simulink model "hikaku"  (R2018b)
settings: Solver=VariableStepAuto  StartTime=0.0  StopTime=3  RelTol=1e-3
values from neighbouring files (symbols this model uses):
  K = lqr(sys_A, sys_B, Q, R)    [LQRadjuster.m]
  L = [0.25; 0.75; -0.15; 0.35]    [LQRadjuster.m]
  x0 = [20*pi/180;0;0;0]    [LQRadjuster.m]
undefined symbols (not defined in the file or in its folder): sys_Ad, sys_Bd, sys_C, sys_D, Ts
settings Model: Creator=kuwano  LastModifiedBy=kuwano

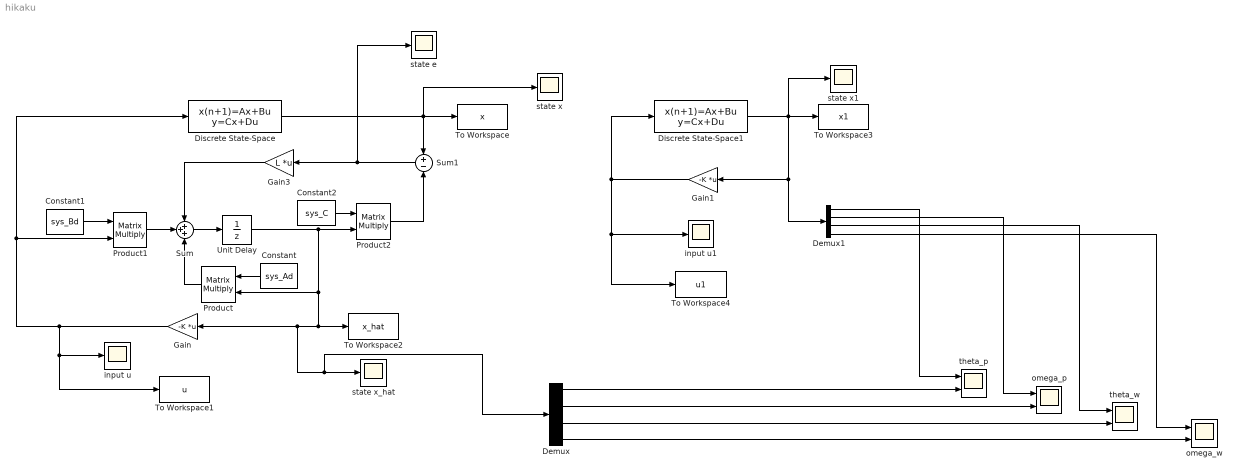
== system hikaku ==
  Constant : Constant  Value=sys_Ad  VectorParams1D=off
  Constant1 : Constant  Value=sys_Bd  VectorParams1D=off
  Constant2 : Constant  Value=sys_C  VectorParams1D=off
  Demux : Demux
  Demux1 : Demux
  Discrete State-Space : DiscreteStateSpace  A=sys_Ad  B=sys_Bd  C=sys_C  D=sys_D  InitialCondition=x0  SampleTime=Ts
  Discrete State-Space1 : DiscreteStateSpace  A=sys_Ad  B=sys_Bd  C=eye(4)  D=[0; 0; 0; 0]  InitialCondition=x0  SampleTime=Ts
  Gain : Gain  Gain=-K  Multiplication=Matrix(K*u)
  Gain1 : Gain  Gain=-K  Multiplication=Matrix(K*u)
  Gain3 : Gain  Gain=L  Multiplication=Matrix(K*u)
  Product : Product  Multiplication=Matrix(*)
  Product1 : Product  Multiplication=Matrix(*)
  Product2 : Product  Multiplication=Matrix(*)
  Sum : Sum  Inputs=+++
  Sum1 : Sum  Inputs=+|-
  To Workspace : ToWorkspace  VariableName=x  SampleTime=-1
  To Workspace1 : ToWorkspace  VariableName=u  SampleTime=-1
  To Workspace2 : ToWorkspace  VariableName=x_hat  SampleTime=-1
  To Workspace3 : ToWorkspace  VariableName=x1  SampleTime=-1
  To Workspace4 : ToWorkspace  VariableName=u1  SampleTime=-1
  Unit Delay : UnitDelay  InitialCondition=[0; 0; 0; 0]  SampleTime=-1
  input u : Scope
  input u1 : Scope
  omega_p : Scope  NumInputPorts=2
  omega_w : Scope  NumInputPorts=2
  state e : Scope
  state x : Scope
  state x1 : Scope
  "state x_hat " : Scope
  theta_p : Scope  NumInputPorts=2
  theta_w : Scope  NumInputPorts=2
  wires:
  Constant1/1 -> Product1/1
  Product/1 -> Sum/3
  Discrete State-Space/1 -> Sum1/1, state x/1, To Workspace/1
  Unit Delay/1 -> Product2/2, Demux/1, "state x_hat "/1, Gain/1, To Workspace2/1, Product/2
  Sum1/1 -> state e/1, Gain3/1
  Constant/1 -> Product/1
  Constant2/1 -> Product2/1
  Product2/1 -> Sum1/2
  Sum/1 -> Unit Delay/1
  Product1/1 -> Sum/2
  Gain/1 -> Discrete State-Space/1, Product1/2, input u/1, To Workspace1/1
  Gain3/1 -> Sum/1
  Discrete State-Space1/1 -> To Workspace3/1, state x1/1, Gain1/1, Demux1/1
  Gain1/1 -> To Workspace4/1, input u1/1, Discrete State-Space1/1
  Demux/4 -> omega_w/2
  Demux1/1 -> theta_p/1
  Demux/1 -> theta_p/2
  Demux1/2 -> omega_p/1
  Demux/2 -> omega_p/2
  Demux/3 -> theta_w/2
  Demux1/4 -> omega_w/1
  Demux1/3 -> theta_w/1
